simulink model "musyndm1"  (Simulink 3.00)
settings: Solver=ode15s  SolverMode=SingleTasking  StartTime=0.0  StopTime=200  RelTol=1e-3  AbsTol=1e-6
PreLoadFcn:
  | mudata1
values from neighbouring files (symbols this model uses):
  a = uperp'*r*vperp'    [ruqvsol.m]    (also in ruqvsolb.m = -[eye(nrr) r1vp;r1vp' eye(ncv-nrv)])
  b = Ueq'*r*vperp'    [ruqvsol.m]    (also in ruqvsolb.m = [zeros(nrr,nrr) r0vp;r0vp' zeros(ncv-nrv,ncv-nrv)])
  bp = pimp(bnum)    [fitchose.m]
  c = uperp'*r*Veq'    [ruqvsol.m]
  cp = cumsum([1;sizecdA(:,1)+sizecdB(:,1)])    [mamilc.m]
  dp = cumsum([1;sizecdA(:,2)+sizecdB(:,2)])    [mamilc.m]
undefined symbols (not defined in the file or in its folder): ak, ap, bk, ck, d, dk
settings Model: ExternalInput=[]  SaveTime=off  SaveOutput=off  InitialState=[]  RTWTemplateMakefile=grt_vc.tmf  ExtModeMexFile=ext_comm.c  Creator=greg  LastModifiedBy=David High

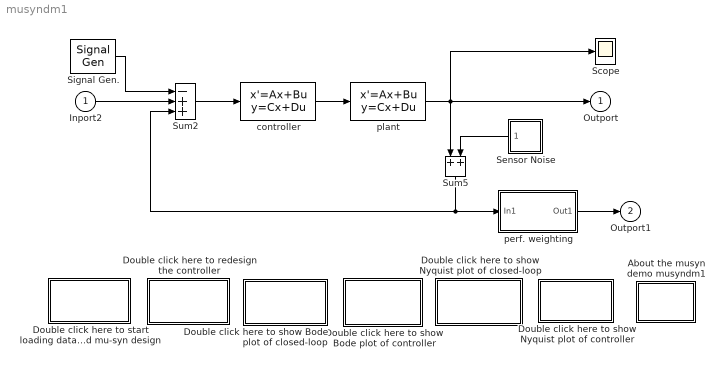
== system musyndm1 ==
  Inport2 : Inport  Port=1  PortWidth=-1  SampleTime=-1  DataType=auto
      settings: SignalType=auto
  About the musyn demo musyndm1 : Subsystem
      settings: OpenFcn=clc; more(24); help mudata1; more off
      mask Display: disp('?')
  Double click here to redesign the controller : Subsystem
      settings: OpenFcn=if ~exist('mu'),fprintf('\nMust be licensed for RCT Toolbox\n'), else, fprintf('\nPress Ctrl_C to abort MuSyn Calculation\n\n'); mudes1; end
      mask Display: disp('Re-design')
  Double click here to show Bode plot of closed-loop : Subsystem
      settings: OpenFcn=if ~exist('mu'),fprintf('\nMust be licensed for Mu Toolbox\n'),elseif ~exist('g1'),fprintf('\nMust Load Data & Design First\n'),else,eval('vplot(''bode'',frsp(g1,logspace(-2,4,32)))');end
      mask Display: disp('Closed-Loop\nBode Plot')
  Double click here to show Bode plot of controller : Subsystem
      settings: OpenFcn=if ~exist('mu'),fprintf('\nMust be licensed for Mu Toolbox\n'),elseif ~exist('k1'),fprintf('\nMust Load Data & Design First\n'),else,eval('vplot(''bode'',frsp(k1,logspace(-2,4,32)))');end
      mask Display: disp('Controller\nBode Plot')
  Double click here to show Nyquist plot of closed-loop : Subsystem
      settings: OpenFcn=if ~exist('mu'),fprintf('\nMust be licensed for Mu Toolbox\n'),elseif ~exist('g1'),fprintf('\nMust Load Data First\n'),else,clf;omtt=logspace(-6,6,100);eval('vplot(''nyq'',frsp(g1,omtt),frsp(g1,-omtt))');end
      mask Display: disp('Closed-Loop\nNyquist')
  Double click here to show Nyquist plot of controller : Subsystem
      settings: OpenFcn=if ~exist('mu'),fprintf('\nMust be licensed for Mu Toolbox\n'),elseif ~exist('g1'),fprintf('\nMust Load Data First\n'),else,clf;omtt=logspace(-6,6,100);eval('vplot(''nyq'',frsp(k1,omtt),frsp(k1,-omtt))');end
      mask Display: disp('Controller\nNyquist')
  Double click here to start loading data and mu-syn design : Subsystem
      settings: OpenFcn=if ~exist('mu'),fprintf('\nMust be licensed for MuSyn Toolbox\n'), else, fprintf('\nLoading Data\nWarning: New data will overlap the original working space data'); mudata1; end
      mask Display: disp('Re-Load\nData')
  Scope : Scope
      settings: TickLabels=on  TimeRange=20.000000  YMin=-5  YMax=5  SaveToWorkspace=off  SaveName=ScopeData  DataFormat=Matrix
  Sensor Noise : Subsystem  Orientation=left  mask{@1=0.02, @2=0.1, @3=[23341]}
      mask prompts: @1 "Noise Power:"; @2 "Sample Time:"; @3 "Seed"
      mask help:
      | White noise for continuous (s-domain) systems.
      | Band-limited using zero-order-hold.
      mask init:
      | Cov = @1; Ts = @2; seed = @3; r = rand(1,12); r2 = [r(1),r;r,r(12)]; t =[1:13;1:13];
      mask Help: Implemented using white noise into Zero-Order Hold block. The seed and power can be vectors of the same length to produce a vector of white noise sources. For faster simulation, set sample time to the highest value possible but in accordance with the fastest dynamics of system.
      mask Display: plot(t(:),r2(:))
  Signal Gen. : SignalGenerator  WaveForm=square  Amplitude=2.000000  Frequency=1.000000  Units=rad/sec
  Sum2 : Sum  Inputs=-++  SaturateOnIntegerOverflow=on
  Sum5 : Sum  Orientation=down  Inputs=++  SaturateOnIntegerOverflow=on
  controller : StateSpace  A=ak  B=bk  C=ck  D=dk  X0=0
  perf. weighting : Subsystem  mask{@1=num, @2=den}
      mask prompts: @1 "numerator:"; @2 "denominator:"
      mask help: Performance weighting function:
      mask init:
      | [ap,bp,cp,dp]=tf2ss(@1,@2);
      mask Help: This is the weighting function of the plant model.
      mask Display: disp('weighting\nfunc.')
  plant : StateSpace  A=a  B=b  C=c  D=d  X0=0
  Outport : Outport  Port=1
  Outport1 : Outport  Port=2
  wires:
  Sum5/1 -> perf. weighting/1(In1), Sum2/3
  Sensor Noise/1(Out_1) -> Sum5/2
  plant/1 -> Scope/1, Sum5/1, Outport/1
  Inport2/1 -> Sum2/2
  perf. weighting/1(Out1) -> Outport1/1
  Signal Gen./1 -> Sum2/1
  Sum2/1 -> controller/1
  controller/1 -> plant/1

== system musyndm1/About the musyn demo musyndm1 ==

== system musyndm1/Double click here to redesign the controller ==

== system musyndm1/Double click here to show Bode plot of closed-loop ==

== system musyndm1/Double click here to show Bode plot of controller ==

== system musyndm1/Double click here to show Nyquist plot of closed-loop ==

== system musyndm1/Double click here to show Nyquist plot of controller ==

== system musyndm1/Double click here to start loading data and mu-syn design ==

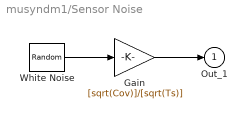
== system musyndm1/Sensor Noise ==
  Gain : Gain  Gain=[sqrt(Cov)]/[sqrt(Ts)]  SaturateOnIntegerOverflow=on
  White Noise : RandomNumber  Mean=0  Variance=1  Seed=seed  SampleTime=Ts
  Out_1 : Outport  Port=1
  wires:
  Gain/1 -> Out_1/1
  White Noise/1 -> Gain/1

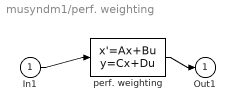
== system musyndm1/perf. weighting ==
  In1 : Inport  Port=1  PortWidth=-1  SampleTime=-1  DataType=auto
      settings: SignalType=auto
  perf. weighting : StateSpace  A=ap  B=bp  C=cp  D=dp  X0=0
  Out1 : Outport  Port=1
  wires:
  In1/1 -> perf. weighting/1
  perf. weighting/1 -> Out1/1
